simulink model "TransientVehicleModel"  (R2026a)
settings: Solver=VariableStepAuto  RelTol=1e-2
values from neighbouring files (symbols this model uses):
  a_ft = a_in * IN2FT    (= 2.62166666667)    [VehicleParameters.m]
  b_ft = b_in * IN2FT    (= 2.42)    [VehicleParameters.m]
  DamperVelocity_in_s = DamperVelocity_mm_s * MMPS2INPS    [VehicleParameters.m]
  DEG2RAD = pi / 180    (= 0.0174532925199)    [VehicleParameters.m]
  FrontRollCenter_ft = FrontRollCenter_in * IN2FT    (= -0.00166666666667)    [VehicleParameters.m]
  FrontRollDamperLever_in = FrontRollMotionRatio * FTrackwidth_in / 2    (= 18.095)    [VehicleParameters.m]
  FrontRollMotionRatio = 0.77    [VehicleParameters.m]
  FrontRollStiffness = 18875    [VehicleParameters.m]
  FrontStaticToe_deg = 0.0    (= 0)    [VehicleParameters.m]
  FrontToeGainHeave_deg_in = 0    [VehicleParameters.m]
  FrontToeGainRoll_deg_deg = 0    [VehicleParameters.m]
  FTrackwidth_ft = FTrackwidth_in * IN2FT    (= 3.91666666667)    [VehicleParameters.m]
  FTrackwidth_in = 47.0    (= 47)    [VehicleParameters.m]
  Gravity = 32.174    [VehicleParameters.m]
  MPH2FPS = 1.46667    [VehicleParameters.m]
  RAD2DEG = 180 / pi    (= 57.2957795131)    [VehicleParameters.m]
  RearRollCenter_ft = RearRollCenter_in * IN2FT    (= 0.206166666667)    [VehicleParameters.m]
  RearRollDamperLever_in = RearRollMotionRatio  * RTrackwidth_in / 2    (= 2.7899)    [VehicleParameters.m]
  RearRollMotionRatio = 0.1213    [VehicleParameters.m]
  RearRollStiffness = 22285    [VehicleParameters.m]
  RearStaticToe_deg = 0.0    (= 0)    [VehicleParameters.m]
  RearToeGainHeave_deg_in = 0    [VehicleParameters.m]
  RearToeGainRoll_deg_deg = 0    [VehicleParameters.m]
  RollInertia_RA = 15.0    (= 15)    [VehicleParameters.m]
  RollMomentArm_ft = CG_ft - RollAxisHeight_ft    (= 0.831093333333)    [VehicleParameters.m]
  RTrackwidth_ft = RTrackwidth_in * IN2FT    (= 3.83333333333)    [VehicleParameters.m]
  SprungMass_slug = SprungMass_lbm * LBM2SLUG    (= 14.3895754336)    [VehicleParameters.m]
  StaticFZ_FL = FrontWeight_lbf / 2    (= 133.335408)    [VehicleParameters.m]
  StaticFZ_FR = FrontWeight_lbf / 2    (= 133.335408)    [VehicleParameters.m]
  StaticFZ_RL = RearWeight_lbf / 2    (= 144.446692)    [VehicleParameters.m]
  StaticFZ_RR = RearWeight_lbf / 2    (= 144.446692)    [VehicleParameters.m]
  TotalMass_slug = TotalMass_lbm * LBM2SLUG    (= 17.2674892771)    [VehicleParameters.m]
  Wheelbase_ft = Wheelbase_in * IN2FT    (= 5.04166666667)    [VehicleParameters.m]
  YawInertia = 67.8557    [VehicleParameters.m]
undefined symbols (not defined in the file or in its folder): Roll
libraries: SignalEditorBlockLib x1
settings Model: Creator=colew  LastModifiedBy=colew

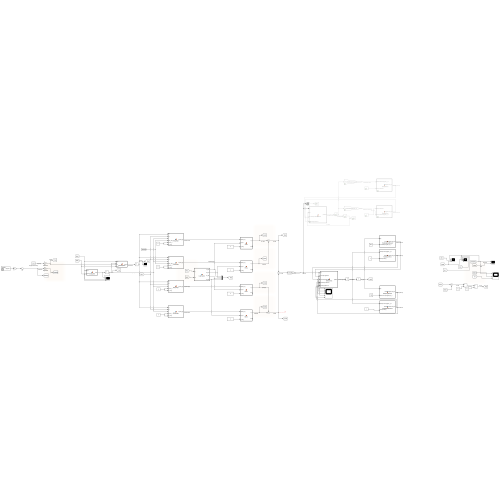
[thumbnail: Simulink's stored preview of the top-level diagram]
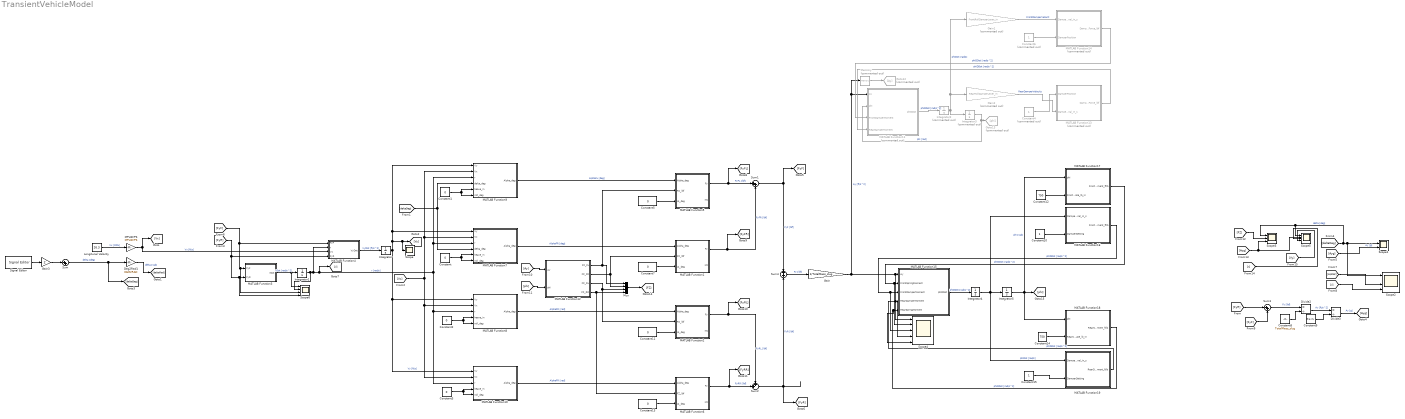
== system TransientVehicleModel ==
  Constant{,1..3,5,7,11,13} (8 alike) : Constant  Value=0
  Constant10 : Constant
  Constant12 : Constant  Value=750
  Constant14 : Constant  Value=750
  Constant15 : Constant
  Constant4 : Constant  Commented=on
  Constant6 : Constant  Commented=on
  Constant8 : Constant  Value=TotalMass_slug
  Constant9 : Constant  Value=Gravity
  Deg2Rad1 : Gain  Gain=DEG2RAD
  Divide2 : Product  Inputs=*/
  Divide3 : Product  Inputs=*/
  Gain : Gain  Gain=1/TotalMass_slug
  Gain1 : Gain  Commented=on  Gain=FrontRollDamperLever_in
  Gain2 : Gain  Commented=on  Gain=RearRollDamperLever_in
  Gain3 : Gain  Gain=2
  Goto12 : Goto  Commented=on  GotoTag=Ay
  Goto13 : Goto  Commented=on  GotoTag=phi
  Integrator{,1,4..5} (4 alike) : Integrator
  Integrator2 : Integrator  Commented=on
  Integrator3 : Integrator  Commented=on
  Longitunal Velocity : Constant  Value=26.3
  MATLAB Function1 : MATLAB Function  TreatAsAtomicUnit=on
  MATLAB Function10 : MATLAB Function  TreatAsAtomicUnit=on
  MATLAB Function11 : MATLAB Function  Commented=on  TreatAsAtomicUnit=on
  MATLAB Function12 : MATLAB Function  TreatAsAtomicUnit=on
  MATLAB Function13 : MATLAB Function  Commented=on  TreatAsAtomicUnit=on
  MATLAB Function14 : MATLAB Function  Commented=on  TreatAsAtomicUnit=on
  MATLAB Function15 : MATLAB Function  TreatAsAtomicUnit=on
  MATLAB Function16 : MATLAB Function  TreatAsAtomicUnit=on
  MATLAB Function17 : MATLAB Function  TreatAsAtomicUnit=on
  MATLAB Function18 : MATLAB Function  TreatAsAtomicUnit=on
  MATLAB Function19 : MATLAB Function  TreatAsAtomicUnit=on
  MATLAB Function2 : MATLAB Function  TreatAsAtomicUnit=on
  MATLAB Function3 : MATLAB Function  TreatAsAtomicUnit=on
  MATLAB Function4 : MATLAB Function  TreatAsAtomicUnit=on
  MATLAB Function5 : MATLAB Function  TreatAsAtomicUnit=on
  MATLAB Function6 : MATLAB Function  TreatAsAtomicUnit=on
  MATLAB Function7 : MATLAB Function  TreatAsAtomicUnit=on
  MATLAB Function8 : MATLAB Function  TreatAsAtomicUnit=on
  MATLAB Function9 : MATLAB Function  TreatAsAtomicUnit=on
  MPH2FPS : Gain  Gain=MPH2FPS
  Memory : Memory  Commented=on
  Mux : Mux
  Scope : Scope
      settings: ActiveDisplayYMinimum=-1  ActiveDisplayYMaximum=1  DataLoggingVariableName=ScopeData3
  Scope1 : Scope  NumInputPorts=2
      settings: ActiveDisplayYMinimum=-0.12499999999999997  ActiveDisplayYMaximum=1.125
  Scope2 : Scope  NumInputPorts=4
      settings: ActiveDisplayYMinimum=-0.12499999999999997  ActiveDisplayYMaximum=1.125
  Scope3 : Scope  NumInputPorts=3
      settings: ActiveDisplayYMinimum=-1.4999999999999996  ActiveDisplayYMaximum=13.5  DataLoggingVariableName=ScopeData2
  Scope4 : Scope  NumInputPorts=5
      settings: ActiveDisplayYMinimum=-1.2900610883905346  ActiveDisplayYMaximum=11.799993396666688  DataLoggingVariableName=ScopeData4
  Scope5 : Scope  NumInputPorts=5
      settings: ActiveDisplayYMinimum=-1.4999999999999996  ActiveDisplayYMaximum=13.5  DataLoggingVariableName=ScopeData5
  Scope6 : Scope  NumInputPorts=4
      settings: ActiveDisplayYMinimum=-0.52606310915248622  ActiveDisplayYMaximum=0.52605923575201241  DataLoggingVariableName=ScopeData6
  Signal Editor : SignalEditorBlockLib/Signal Editor  FileName=C:\Users\colew\Documents\FSAE\FSAE-VD\MatLab\Signals\0-1-0gental  ActiveScenario=Scenario  ActiveSignal=Signal 1  IsBus=off  OutputBusObjectStr=Bus: BusObject  SampleTime=0  ZeroCross=off  OutputAfterFinalValue=Setting to zero  Unit=inherit  PreserveSignalName=on  ApplySigPropsToAllScenarios=on  ApplySigPropsToAllSignals=off  SignalPropertySource=Dialog parameters
  Sum : Sum  Inputs=|++
  Sum1 : Sum  Inputs=|++
  Sum2 : Sum  Inputs=++|
  Sum3 : Sum  Inputs=|++
  Sum4 : Sum
  wires:
  Longitunal Velocity/1 -> MPH2FPS/1  "Vx [MPH]"
  Sum/1 -> [deltaDeg], Deg2Rad1/1  "delta [deg]"
  MATLAB Function4/1(VyDot) -> Integrator/1  "VyDot [ft/s^2]"
  MATLAB Function3/1(rDot) -> Scope6/1, Integrator1/1  "rDot [rad/s^2]"
  Integrator/1 -> MATLAB Function7/1(Vy), MATLAB Function9/1(Vy), Scope/1, [Vy], MATLAB Function10/1(Vy), MATLAB Function8/1(Vy)  "Vy [ft/s]"
  MPH2FPS/1 -> MATLAB Function4/3(Vx), [Vx]  "Vx [ft/s]"
  Deg2Rad1/1 -> [deltaRad]  "delta [rad]"
  MATLAB Function7/1(Alpha_deg) -> MATLAB Function1/1(Alpha_deg)  "AlphaFR [deg]"
  Sum3/1 -> Divide2/1  "Fy [lbf]"
  Constant8/1 -> Divide2/2
  Divide2/1 -> Divide3/1  "Ay [ft/s^2]"
  Constant9/1 -> Divide3/2
  Divide3/1 -> [Ayg]  "Ay [g]"
  [deltaDeg] -> Scope5/1, Scope3/1, Scope2/1, Scope1/1  "delta [deg]"
  [Ayg] -> Scope1/2  "Ay [g]"
  [AlphaF] -> Scope2/3
  [r] -> Scope2/4
  [deltaDeg] -> MATLAB Function9/4(delta_deg), MATLAB Function7/4(delta_deg)
  Constant/1 -> MATLAB Function7/5(heave_in), MATLAB Function7/6(roll_deg)
  Integrator1/1 -> Scope6/2, MATLAB Function10/3(r), MATLAB Function8/3(r), MATLAB Function7/3(r), MATLAB Function9/3(r), [r], MATLAB Function4/2(r)  "r [rad/s]"
  [Vx] -> MATLAB Function8/2(Vx), MATLAB Function10/2(Vx), MATLAB Function7/2(Vx), MATLAB Function9/2(Vx)
  MATLAB Function9/1(Alpha_deg) -> MATLAB Function5/1(Alpha_deg)  "AlphaFL [deg]"
  Constant1/1 -> MATLAB Function9/6(roll_deg), MATLAB Function9/5(heave_in)
  Constant2/1 -> MATLAB Function8/4(heave_in), MATLAB Function8/5(roll_deg)
  Constant3/1 -> MATLAB Function10/4(heave_in), MATLAB Function10/5(roll_deg)
  MATLAB Function8/1(Alpha_deg) -> MATLAB Function2/1(Alpha_deg)  "AlphaFR [rad]"
  MATLAB Function10/1(Alpha_deg) -> MATLAB Function6/1(Alpha_deg)  "AlphaFR [rad]"
  MATLAB Function5/1(Fy) -> [FyFL], Sum1/1  "FyFL [lbf]"
  MATLAB Function1/1(Fy) -> [FyFR], Sum1/2  "FyFR [lbf]"
  MATLAB Function6/1(Fy) -> [FyRR], Sum2/2  "FyRR [lbf]"
  MATLAB Function2/1(Fy) -> [FyRL], Sum2/1  "FyRL [lbf]"
  Sum2/1 -> [FyR], Sum4/2  "FyR [lbf]"
  Sum1/1 -> Sum4/1, [FyF]  "FyF [lbf]"
  [FyR] -> MATLAB Function4/4(FyR), Scope6/4, MATLAB Function3/2(FyR)
  [FyF] -> MATLAB Function4/1(FyF), Scope6/3, MATLAB Function3/1(FyF)
  [FyR] -> Sum3/1
  [FyF] -> Sum3/2
  Constant5/1 -> MATLAB Function5/3(IA_deg)
  Constant7/1 -> MATLAB Function1/3(IA_deg)
  Constant11/1 -> MATLAB Function2/3(IA_deg)
  Constant13/1 -> MATLAB Function6/3(IA_deg)
  Sum4/1 -> Gain/1  "Fy [lbf]"
  Gain/1 -> Scope4/1, MATLAB Function15/1(Ay), MATLAB Function11/1(Ay), Memory/1  "Ay [ft/s^2]"
  MATLAB Function11/1(phiDDot) -> Integrator2/1  "phiDDot [rad/s^2]"
  Integrator2/1 -> Integrator3/1, Gain1/1, Gain2/1  "phiDot [rad/s]"
  Integrator3/1 -> Goto13/1, MATLAB Function11/2(phi)  "phi [rad]"
  [Ay] -> MATLAB Function12/1(Ay)
  [phi] -> MATLAB Function12/2(phi)
  Memory/1 -> Goto12/1
  MATLAB Function12/1(FZ_FL) -> Mux/1, MATLAB Function5/2(FZ_lbf)
  MATLAB Function12/2(FZ_FR) -> MATLAB Function1/2(FZ_lbf), Mux/2
  MATLAB Function12/4(FZ_RR) -> MATLAB Function6/2(FZ_lbf), Mux/4
  MATLAB Function12/3(FZ_RL) -> Mux/3, MATLAB Function2/2(FZ_lbf)
  Mux/1 -> [FZ]
  [FZ] -> Scope3/2
  Gain1/1 -> MATLAB Function14/1(DamperVelocitySignal_in_s)  "FrontDamperVelocit"
  Gain2/1 -> MATLAB Function13/2(DamperVelocitySignal_in_s)  "RearDamperVelocity"
  Constant4/1 -> MATLAB Function13/1(DamperPosition)
  Constant6/1 -> MATLAB Function14/2(DamperPosition)
  MATLAB Function14/1(DamperForce_lbf) -> MATLAB Function11/3(FrontDamperMoment)  "phiDDot [rad/s^2]"
  MATLAB Function13/1(DamperForce_lbf) -> MATLAB Function11/4(RearDamperMoment)  "phiDDot [rad/s^2]"
  MATLAB Function15/1(phiDDot) -> Integrator4/1  "phiDDot [rad/s^2]"
  Integrator4/1 -> MATLAB Function19/1(DamperVelocitySignal_in_s), MATLAB Function16/1(DamperVelocitySignal_in_s), Integrator5/1  "phiDot [rad/s]"
  Integrator5/1 -> MATLAB Function18/1(phi), MATLAB Function17/1(phi), [phi]  "phi [rad]"
  Constant10/1 -> MATLAB Function16/2(DamperSetting)
  Constant12/1 -> MATLAB Function17/2(FrontRollSpringRate_lb_in)
  MATLAB Function16/1(FrontDamperMoment_ftlb) -> Scope4/3, MATLAB Function15/3(FrontDamperMoment)  "phiDDot [rad/s^2]"
  MATLAB Function17/1(FrontSpringMoment_ftlb) -> Scope4/2, MATLAB Function15/2(FrontSpringMoment)  "phiDDot [rad/s^2]"
  Constant14/1 -> MATLAB Function18/2(RearCornerSpringRate_lb_in)
  Constant15/1 -> MATLAB Function19/2(DamperSetting)
  MATLAB Function19/1(RearDamperMoment_ftlb) -> Scope4/4, MATLAB Function15/4(RearDamperMoment)  "phiDDot [rad/s^2]"
  MATLAB Function18/1(RearSpringMoment_ftlb) -> Scope4/5, MATLAB Function15/5(RearSpringMoment)  "phiDDot [rad/s^2]"
  [Ayg] -> Scope3/3, Scope5/2
  Gain3/1 -> Sum/1
  Signal Editor/1 -> Gain3/1
  [r] -> Scope5/3
  [Vy] -> Scope5/4

== matlab function TransientVehicleModel/MATLAB Function7 ==
  data: Vy input; Alpha_deg output; Vx input; r input; delta_deg input; a_ft parameter; FTrackwidth_ft parameter; heave_in input; roll_deg input; FrontStaticToe_deg parameter; FrontToeGainRoll_deg_deg parameter; FrontToeGainHeave_deg_in parameter; RAD2DEG parameter
function Alpha_deg = FRSlipAngle(Vy, Vx, r, delta_deg, a_ft, FTrackwidth_ft, heave_in, roll_deg, FrontStaticToe_deg, FrontToeGainRoll_deg_deg, FrontToeGainHeave_deg_in, RAD2DEG)

Steering = delta_deg - (FrontToeGainRoll_deg_deg * roll_deg) - (FrontToeGainHeave_deg_in * heave_in) - FrontStaticToe_deg;

Alpha_deg = Steering - (RAD2DEG * atan((Vy + a_ft*r)/(Vx + r*FTrackwidth_ft/2)));

end

== matlab function TransientVehicleModel/MATLAB Function8 ==
  data: Vy input; Alpha_deg output; Vx input; r input; RTrackwidth_ft parameter; heave_in input; roll_deg input; RAD2DEG parameter; b_ft parameter; RearStaticToe_deg parameter; RearToeGainRoll_deg_deg parameter; RearToeGainHeave_deg_in parameter
function Alpha_deg = RLSlipAngle(Vy, Vx, r, RTrackwidth_ft, heave_in, roll_deg, RAD2DEG, b_ft, RearStaticToe_deg, RearToeGainRoll_deg_deg, RearToeGainHeave_deg_in)

Toe_deg = RearStaticToe_deg + (RearToeGainRoll_deg_deg * roll_deg) + (RearToeGainHeave_deg_in * heave_in);

Alpha_deg = Toe_deg - (RAD2DEG * atan((Vy - b_ft*r)/(Vx - r*RTrackwidth_ft/2)));

end

== matlab function TransientVehicleModel/MATLAB Function9 ==
  data: Vy input; Alpha_deg output; Vx input; r input; delta_deg input; a_ft parameter; FTrackwidth_ft parameter; heave_in input; roll_deg input; FrontStaticToe_deg parameter; FrontToeGainRoll_deg_deg parameter; FrontToeGainHeave_deg_in parameter; RAD2DEG parameter
function Alpha_deg = FLSlipAngle(Vy, Vx, r, delta_deg, a_ft, FTrackwidth_ft, heave_in, roll_deg, FrontStaticToe_deg, FrontToeGainRoll_deg_deg, FrontToeGainHeave_deg_in, RAD2DEG)

Steering = delta_deg + (FrontToeGainRoll_deg_deg * roll_deg) + (FrontToeGainHeave_deg_in * heave_in) + FrontStaticToe_deg;

Alpha_deg = Steering - (RAD2DEG * atan((Vy + a_ft * r)/(Vx - r * FTrackwidth_ft / 2)));

end

== matlab function TransientVehicleModel/MATLAB Function10 ==
  data: Vy input; Alpha_deg output; Vx input; r input; RTrackwidth_ft parameter; heave_in input; roll_deg input; RAD2DEG parameter; RearStaticToe_deg parameter; b_ft parameter; RearToeGainRoll_deg_deg parameter; RearToeGainHeave_deg_in parameter
function Alpha_deg = RRSlipAngle(Vy, Vx, r, RTrackwidth_ft, heave_in, roll_deg, RAD2DEG, RearStaticToe_deg, b_ft, RearToeGainRoll_deg_deg, RearToeGainHeave_deg_in)

Toe_deg = -RearStaticToe_deg - (RearToeGainRoll_deg_deg * roll_deg) - (RearToeGainHeave_deg_in * heave_in);

Alpha_deg = Toe_deg - (RAD2DEG * atan((Vy - b_ft*r)/(Vx + r*RTrackwidth_ft/2)));

end

== matlab function TransientVehicleModel/MATLAB Function11 ==
  data: Ay input; phiDDot output; phi input; FrontDamperMoment input; RearDamperMoment input; RollInertia_RA parameter; SprungMass_slug parameter; RollMomentArm_ft parameter; RearRollStiffness parameter; FrontRollStiffness parameter
function phiDDot = RollDynamics(Ay, phi, FrontDamperMoment, RearDamperMoment, RollInertia_RA, SprungMass_slug, RollMomentArm_ft, RearRollStiffness, FrontRollStiffness)

% Lateral acceleration trying to roll the car
RollMoment = SprungMass_slug * Ay * RollMomentArm_ft;

% Springs resisting roll
FrontSpringMoment = FrontRollStiffness * phi;
RearSpringMoment  = RearRollStiffness  * phi;

% Sum moments about roll axis
NetMoment = RollMoment - FrontSpringMoment - RearSpringMoment + FrontDamperMoment + RearDamperMoment;

% Roll acceleration
phiDDot = NetMoment / RollInertia_RA;

end

== matlab function TransientVehicleModel/MATLAB Function12 ==
  data: Ay input; FZ_FL output; FZ_FR output; FZ_RL output; phi input; SprungMass_slug parameter; Wheelbase_ft parameter; FrontRollCenter_ft parameter; FrontRollStiffness parameter; RearRollStiffness parameter; FZ_RR output; RearRollCenter_ft parameter; FTrackwidth_ft parameter; RTrackwidth_ft parameter; StaticFZ_FL parameter; StaticFZ_FR parameter; StaticFZ_RL parameter; StaticFZ_RR parameter; a_ft parameter; b_ft parameter
function [FZ_FL, FZ_FR, FZ_RL, FZ_RR]  = LoadTransfer(Ay, phi, SprungMass_slug, Wheelbase_ft, FrontRollCenter_ft, FrontRollStiffness, RearRollStiffness, RearRollCenter_ft, FTrackwidth_ft, RTrackwidth_ft, StaticFZ_FL, StaticFZ_FR, StaticFZ_RL, StaticFZ_RR, a_ft, b_ft)

% Sprung-mass lateral force
Ys = SprungMass_slug * Ay;

% Lateral force distribution
YF = Ys * b_ft / Wheelbase_ft;
YR = Ys * a_ft / Wheelbase_ft;

% Geometric roll moments
FrontGeoMoment = YF * FrontRollCenter_ft;
RearGeoMoment  = YR * RearRollCenter_ft;

% Elastic roll moments
FrontElasticMoment = FrontRollStiffness * phi;
RearElasticMoment  = RearRollStiffness * phi;

% Total axle roll moments
FrontRollMoment = FrontGeoMoment + FrontElasticMoment;
RearRollMoment  = RearGeoMoment  + RearElasticMoment;

% Load transfer
FrontLoadTransfer = FrontRollMoment / FTrackwidth_ft;
RearLoadTransfer  = RearRollMoment  / RTrackwidth_ft;

% Tire vertical loads
FZ_FL = StaticFZ_FL - FrontLoadTransfer;
FZ_FR = StaticFZ_FR + FrontLoadTransfer;

FZ_RL = StaticFZ_RL - RearLoadTransfer;
FZ_RR = StaticFZ_RR + RearLoadTransfer;

end

== matlab function TransientVehicleModel/MATLAB Function13 ==
  data: DamperPosition input; Roll parameter; DamperForce_lbf output; DamperVelocitySignal_in_s input; DamperVelocity_in_s parameter
function DamperForce_lbf = RollDamperForce(DamperPosition, Roll, DamperVelocitySignal_in_s, DamperVelocity_in_s)

% Convert physical position 0-11 to MATLAB column 1-12
Column = round(DamperPosition) + 1;
Column = min(max(Column,1),12);

% Selected VC01 force curve
ForceCurve = Roll.VC01.Compression_lbf(:,Column);

% Current damper speed
Speed = abs(DamperVelocitySignal_in_s);

% Lookup tables
VelocityTable = [0; DamperVelocity_in_s(:)];
ForceTable = [0; ForceCurve(:)];

% Interpolate
ForceMagnitude = interp1( ...
    VelocityTable, ...
    ForceTable, ...
    Speed, ...
    'linear', ...
    'extrap');

% Damper opposes motion
DamperForce_lbf = ...
    -sign(DamperVelocitySignal_in_s) * ForceMagnitude;

end

== matlab function TransientVehicleModel/MATLAB Function14 ==
  data: DamperVelocitySignal_in_s input; DamperForce_lbf output; DamperPosition input; Roll parameter; DamperVelocity_in_s parameter
function DamperForce_lbf = RollDamperForce(DamperVelocitySignal_in_s, DamperPosition, Roll, DamperVelocity_in_s)

% Convert physical position 0-11 to MATLAB column 1-12
Column = round(DamperPosition) + 1;
Column = min(max(Column,1),12);

% Selected VC01 force curve
ForceCurve = Roll.VC01.Compression_lbf(:,Column);

% Current damper speed
Speed = abs(DamperVelocitySignal_in_s);

% Lookup tables
VelocityTable = [0; DamperVelocity_in_s(:)];
ForceTable = [0; ForceCurve(:)];

% Interpolate
ForceMagnitude = interp1( ...
    VelocityTable, ...
    ForceTable, ...
    Speed, ...
    'linear', ...
    'extrap');

% Damper opposes motion
DamperForce_lbf = ...
    -sign(DamperVelocitySignal_in_s) * ForceMagnitude;

end

== matlab function TransientVehicleModel/MATLAB Function15 ==
  data: Ay input; phiDDot output; FrontSpringMoment input; FrontDamperMoment input; RearDamperMoment input; RollInertia_RA parameter; SprungMass_slug parameter; RollMomentArm_ft parameter; RearSpringMoment input
function phiDDot = RollDynamics(Ay, FrontSpringMoment, FrontDamperMoment, RearDamperMoment, RollInertia_RA, SprungMass_slug, RollMomentArm_ft, RearSpringMoment)

% Lateral acceleration trying to roll the car

RollMoment = SprungMass_slug * Ay * RollMomentArm_ft;

% Sum moments about roll axis

NetMoment = RollMoment + FrontSpringMoment + RearSpringMoment + FrontDamperMoment + RearDamperMoment;

% Roll acceleration

phiDDot = NetMoment / RollInertia_RA;

end

== matlab function TransientVehicleModel/MATLAB Function16 ==
  data: DamperVelocitySignal_in_s input; DamperSetting input; FrontDamperMoment_ftlb output; Roll parameter; DamperVelocity_in_s parameter; FrontRollMotionRatio parameter; FTrackwidth_ft parameter
function FrontDamperMoment_ftlb = RollDamperForce(DamperVelocitySignal_in_s, DamperSetting, Roll, DamperVelocity_in_s, FrontRollMotionRatio, FTrackwidth_ft)

% Convert physical position 0-11 to MATLAB column 1-12
Column = round(DamperSetting) + 1;
Column = min(max(Column,1),12);

% Selected VC01 force curve
ForceCurve = Roll.VC01.Compression_lbf(:,Column);

% Current damper speed
Speed = abs(DamperVelocitySignal_in_s);

% Lookup tables
VelocityTable = [0; DamperVelocity_in_s(:)];
ForceTable = [0; ForceCurve(:)];

% Interpolate
ForceMagnitude = interp1( ...
    VelocityTable, ...
    ForceTable, ...
    Speed, ...
    'linear', ...
    'extrap');

% Damper opposes motion
DamperForce_lbf = -sign(DamperVelocitySignal_in_s) * ForceMagnitude;

% Effective roll lever arm at the damper
LeverArm_ft = FrontRollMotionRatio * (FTrackwidth_ft / 2);

% Damper roll moment
FrontDamperMoment_ftlb = DamperForce_lbf * LeverArm_ft;

end

== matlab function TransientVehicleModel/MATLAB Function17 ==
  data: phi input; FrontSpringMoment_ftlb output; FrontRollSpringRate_lb_in input; FrontRollMotionRatio parameter; FTrackwidth_in parameter
function FrontSpringMoment_ftlb = FrontRollSpringMoment(phi, FrontRollSpringRate_lb_in, FrontRollMotionRatio, FTrackwidth_in)

% Effective front roll stiffness
% Output units: lbf*ft/rad

FrontRollStiffness_ftlb_rad = ...
    FrontRollSpringRate_lb_in ...
    * FrontRollMotionRatio^2 ...
    * FTrackwidth_in^2 ...
    / (4 * 12);

% Spring opposes roll

FrontSpringMoment_ftlb = ...
    -FrontRollStiffness_ftlb_rad * phi;

end

== matlab function TransientVehicleModel/MATLAB Function18 ==
  data: phi input; RearCornerSpringRate_lb_in input; RearSpringMoment_ftlb output; RearRollMotionRatio parameter; RTrackwidth_ft parameter
function RearSpringMoment_ftlb = RearSpringMoment(phi, RearCornerSpringRate_lb_in, RearRollMotionRatio, RTrackwidth_ft)

% One rear wheel vertical displacement from chassis roll
WheelDisplacement_ft = phi * (RTrackwidth_ft / 2);

% Convert wheel displacement to spring displacement
SpringDisplacement_in = WheelDisplacement_ft * 12 * RearRollMotionRatio;

% Force from ONE rear spring
SpringForce_lbf = -RearCornerSpringRate_lb_in * SpringDisplacement_in;

% Effective lever arm of ONE spring about roll axis
LeverArm_ft = RearRollMotionRatio * (RTrackwidth_ft / 2);

% Both rear springs resist roll
RearSpringMoment_ftlb = 2 * SpringForce_lbf * LeverArm_ft;

end

== matlab function TransientVehicleModel/MATLAB Function19 ==
  data: DamperVelocitySignal_in_s input; RearDamperMoment_ftlb output; RearRollMotionRatio parameter; RTrackwidth_ft parameter; Roll parameter; DamperVelocity_in_s parameter; DamperSetting input
function RearDamperMoment_ftlb  = RearRollDamperForce( ...
    DamperVelocitySignal_in_s, ...
    RearRollMotionRatio, ...
    RTrackwidth_ft, Roll, ...
DamperVelocity_in_s, ...
DamperSetting) ...

% Convert physical position 0-11 to MATLAB column 1-12

Column = round(DamperSetting) + 1;

Column = min(max(Column,1),12);

% Use the SAME VC01 force curve as the front

ForceCurve = Roll.VC01.Compression_lbf(:,Column);

% Current damper speed

Speed = abs(DamperVelocitySignal_in_s);

% Same lookup tables as front

VelocityTable = [0; DamperVelocity_in_s(:)];

ForceTable = [0; ForceCurve(:)];

% Interpolate

ForceMagnitude = interp1( ...
    VelocityTable, ...
    ForceTable, ...
    Speed, ...
    'linear', ...
    'extrap');

% Damper opposes motion

DamperForce_lbf = ...
    -sign(DamperVelocitySignal_in_s) * ForceMagnitude;

% Effective lever arm for ONE rear corner damper

LeverArm_ft = ...
    RearRollMotionRatio * (RTrackwidth_ft / 2);

% TWO rear dampers contribute to roll

RearDamperMoment_ftlb = ...
    2 * DamperForce_lbf * LeverArm_ft;

end

== matlab function TransientVehicleModel/MATLAB Function1 ==
  data: Alpha_deg input; Fy output; FZ_lbf input; IA_deg input; Mz output; Tire parameter
function [Fy, Mz] = FRTire(Alpha_deg, FZ_lbf, IA_deg, Tire)

%% INPUT CONVERSIONS

ALPHA = Alpha_deg * pi/180;
GAMMA = IA_deg * pi/180;

FZ0 = Tire.FNOMIN_lbf * Tire.LFZO;
DFZ = (FZ_lbf - FZ0) / FZ0;


%% LATERAL FORCE

GAMY = GAMMA * Tire.LGAY;

SHY = (Tire.PHY1 + Tire.PHY2*DFZ + Tire.PHY3*GAMY) * Tire.LHY;

ALPHAY = ALPHA + SHY;

SVY = FZ_lbf * ((Tire.PVY1 + Tire.PVY2*DFZ) + (Tire.PVY3 + Tire.PVY4*DFZ)*GAMY) * Tire.LVY * Tire.LMUY;

CY = Tire.PCY1 * Tire.LCY;

MUY = (Tire.PDY1 + Tire.PDY2*DFZ) * (1 - Tire.PDY3*GAMY^2) * Tire.LMUY;

DY = MUY * FZ_lbf;

KY = Tire.PKY1 * FZ0 * sin(2*atan(FZ_lbf/(Tire.PKY2*FZ0))) * (1 - Tire.PKY3*abs(GAMY)) * Tire.LKY;

BY = KY / (CY*DY + 1e-9);

EY = (Tire.PEY1 + Tire.PEY2*DFZ) * (1 - (Tire.PEY3 + Tire.PEY4*GAMY)*sign(ALPHAY)) * Tire.LEY;

Fy = DY * sin(CY*atan(BY*ALPHAY - EY*(BY*ALPHAY - atan(BY*ALPHAY)))) + SVY;


%% ALIGNING MOMENT

Mz = 0;

end

== matlab function TransientVehicleModel/MATLAB Function2 ==
  data: Alpha_deg input; Fy output; FZ_lbf input; IA_deg input; Mz output; Tire parameter
function [Fy, Mz] = RLTire(Alpha_deg, FZ_lbf, IA_deg, Tire)

%% INPUT CONVERSIONS

ALPHA = Alpha_deg * pi/180;
GAMMA = IA_deg * pi/180;

FZ0 = Tire.FNOMIN_lbf * Tire.LFZO;
DFZ = (FZ_lbf - FZ0) / FZ0;


%% LATERAL FORCE

GAMY = GAMMA * Tire.LGAY;

SHY = (Tire.PHY1 + Tire.PHY2*DFZ + Tire.PHY3*GAMY) * Tire.LHY;

ALPHAY = ALPHA + SHY;

SVY = FZ_lbf * ((Tire.PVY1 + Tire.PVY2*DFZ) + (Tire.PVY3 + Tire.PVY4*DFZ)*GAMY) * Tire.LVY * Tire.LMUY;

CY = Tire.PCY1 * Tire.LCY;

MUY = (Tire.PDY1 + Tire.PDY2*DFZ) * (1 - Tire.PDY3*GAMY^2) * Tire.LMUY;

DY = MUY * FZ_lbf;

KY = Tire.PKY1 * FZ0 * sin(2*atan(FZ_lbf/(Tire.PKY2*FZ0))) * (1 - Tire.PKY3*abs(GAMY)) * Tire.LKY;

BY = KY / (CY*DY + 1e-9);

EY = (Tire.PEY1 + Tire.PEY2*DFZ) * (1 - (Tire.PEY3 + Tire.PEY4*GAMY)*sign(ALPHAY)) * Tire.LEY;

Fy = DY * sin(CY*atan(BY*ALPHAY - EY*(BY*ALPHAY - atan(BY*ALPHAY)))) + SVY;


%% ALIGNING MOMENT

Mz = 0;

end

== matlab function TransientVehicleModel/MATLAB Function3 ==
  data: FyF input; rDot output; FyR input; a_ft parameter; b_ft parameter; YawInertia parameter
function rDot = YawEquation(FyF, FyR, a_ft, b_ft, YawInertia)

rDot = (a_ft*FyF - b_ft*FyR)/YawInertia;

end

== matlab function TransientVehicleModel/MATLAB Function4 ==
  data: FyF input; r input; VyDot output; Vx input; FyR input; TotalMass_slug parameter
function VyDot = LateralEquation(FyF, r, Vx, FyR, TotalMass_slug)

VyDot = (FyF + FyR)/TotalMass_slug - Vx*r;

end

== matlab function TransientVehicleModel/MATLAB Function5 ==
  data: Alpha_deg input; Fy output; FZ_lbf input; IA_deg input; Mz output; Tire parameter
function [Fy, Mz] = FLTire(Alpha_deg, FZ_lbf, IA_deg, Tire)

%% INPUT CONVERSIONS

ALPHA = Alpha_deg * pi/180;
GAMMA = IA_deg * pi/180;

FZ0 = Tire.FNOMIN_lbf * Tire.LFZO;
DFZ = (FZ_lbf - FZ0) / FZ0;


%% LATERAL FORCE

GAMY = GAMMA * Tire.LGAY;

SHY = (Tire.PHY1 + Tire.PHY2*DFZ + Tire.PHY3*GAMY) * Tire.LHY;

ALPHAY = ALPHA + SHY;

SVY = FZ_lbf * ((Tire.PVY1 + Tire.PVY2*DFZ) + (Tire.PVY3 + Tire.PVY4*DFZ)*GAMY) * Tire.LVY * Tire.LMUY;

CY = Tire.PCY1 * Tire.LCY;

MUY = (Tire.PDY1 + Tire.PDY2*DFZ) * (1 - Tire.PDY3*GAMY^2) * Tire.LMUY;

DY = MUY * FZ_lbf;

KY = Tire.PKY1 * FZ0 * sin(2*atan(FZ_lbf/(Tire.PKY2*FZ0))) * (1 - Tire.PKY3*abs(GAMY)) * Tire.LKY;

BY = KY / (CY*DY + 1e-9);

EY = (Tire.PEY1 + Tire.PEY2*DFZ) * (1 - (Tire.PEY3 + Tire.PEY4*GAMY)*sign(ALPHAY)) * Tire.LEY;

Fy = DY * sin(CY*atan(BY*ALPHAY - EY*(BY*ALPHAY - atan(BY*ALPHAY)))) + SVY;


%% ALIGNING MOMENT

% Add validated MF5.2 MZ equation here next.

Mz = 0;

end

== matlab function TransientVehicleModel/MATLAB Function6 ==
  data: Alpha_deg input; Fy output; FZ_lbf input; IA_deg input; Mz output; Tire parameter
function [Fy, Mz] = RRTire(Alpha_deg, FZ_lbf, IA_deg, Tire)

%% INPUT CONVERSIONS

ALPHA = Alpha_deg * pi/180;
GAMMA = IA_deg * pi/180;

FZ0 = Tire.FNOMIN_lbf * Tire.LFZO;
DFZ = (FZ_lbf - FZ0) / FZ0;


%% LATERAL FORCE

GAMY = GAMMA * Tire.LGAY;

SHY = (Tire.PHY1 + Tire.PHY2*DFZ + Tire.PHY3*GAMY) * Tire.LHY;

ALPHAY = ALPHA + SHY;

SVY = FZ_lbf * ((Tire.PVY1 + Tire.PVY2*DFZ) + (Tire.PVY3 + Tire.PVY4*DFZ)*GAMY) * Tire.LVY * Tire.LMUY;

CY = Tire.PCY1 * Tire.LCY;

MUY = (Tire.PDY1 + Tire.PDY2*DFZ) * (1 - Tire.PDY3*GAMY^2) * Tire.LMUY;

DY = MUY * FZ_lbf;

KY = Tire.PKY1 * FZ0 * sin(2*atan(FZ_lbf/(Tire.PKY2*FZ0))) * (1 - Tire.PKY3*abs(GAMY)) * Tire.LKY;

BY = KY / (CY*DY + 1e-9);

EY = (Tire.PEY1 + Tire.PEY2*DFZ) * (1 - (Tire.PEY3 + Tire.PEY4*GAMY)*sign(ALPHAY)) * Tire.LEY;

Fy = DY * sin(CY*atan(BY*ALPHAY - EY*(BY*ALPHAY - atan(BY*ALPHAY)))) + SVY;


%% ALIGNING MOMENT

Mz = 0;

end
